simulink model "untitled"  (R2023a)
settings: Solver=VariableStepAuto  StartTime=0  StopTime=1435  RelTol=1e-3
libraries: autolibshared x1
settings Model: Creator=Leviathan  LastModifiedBy=Leviathan

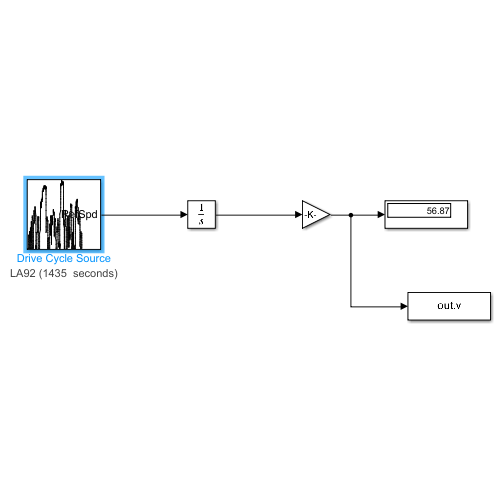
[thumbnail: Simulink's stored preview of the top-level diagram]
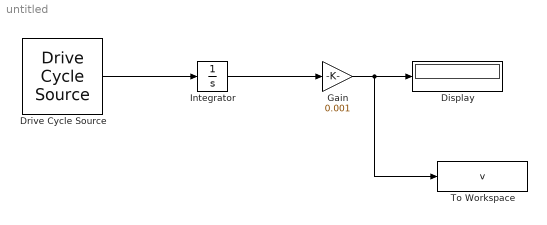
== system untitled ==
  Display : Display
  Drive Cycle Source : autolibshared/Drive Cycle Source  cycleVar=LA92  fileVar=C:\Users\Leviathan\Desktop\WLTC工况.xlsx  tfinal="1435  seconds"  cycleRepeat=off  outAccPort=off  outGearPort=off  gearList=No gear data  t_wot1=1  xdot_woto=0  xdot_wot1=26.8  t_wot2=30  xdot_wot2=0  t_wotend=40  srcUnit=m/s  outUnit=km/h  srcAccUnit=m/s/s  outAccUnit=m/s^2  dt=0  aMode=1  faultOption=off  velBnd=2  velBndUnit=mph  inUnit=m/s  timeBnd=1  failOption=off  stopSim=off  maxFaultCnt=10  maxFaultTime=2  maxTotFaultTime=15  traceOption=off  dtTrace=1  traceWindow=10  lastDCname=LA92  lastOutUnit=mph  lastDT=0  lastTB=1  lastSB=2  forceCalcBound=off
  Gain : Gain  Gain=0.001
  Integrator : Integrator
  To Workspace : ToWorkspace  VariableName=v  SampleTime=1
  wires:
  Drive Cycle Source/1 -> Integrator/1
  Integrator/1 -> Gain/1
  Gain/1 -> To Workspace/1, Display/1
